simulink model "mp_rl_load_class"  (R2021b)
settings: Solver=ode23tb  StartTime=0.0  StopTime=0.1  RelTol=1e-3
values from neighbouring files (symbols this model uses):
  A = -R/L    (= -200)    [init_mp_rl_load.m]    (also in init_mp_rl_load_class.m = 0.99)
  Atilde = -R/L    (= -1000)    [init_mp_rl_load_class.m]
  B = 1/L    (= 200)    [init_mp_rl_load.m]    (also in init_mp_rl_load_class.m = 0.01)
  Btilde = 1/L    (= 1000)    [init_mp_rl_load_class.m]
  C = 1    [init_mp_rl_load.m]    (also in init_mp_rl_load_class.m)
  i_ref_amp = 50    [init_mp_rl_load_class.m]
  i_ref_omega = 2*pi*50    (= 314.159265359)    [init_mp_rl_load_class.m]
  rho = 0    [init_mp_rl_load.m]    (also in init_mp_rl_load_class.m = 0.0001)
  ts = 1e-5    (= 1e-05)    [init_mp_rl_load_class.m]
  udc = 250    [init_mp_rl_load.m]    (also in init_mp_rl_load_class.m)
settings Model: Creator=dbagn  LastModifiedBy=dbagn
settings SolverCC: AlgebraicLoopSolver=TrustRegion
settings DebuggingCC: SFMachineParentedDataDiag=warning
settings SFSimCC: CustomCodeUndefinedFunction=UseInterfaceOnly

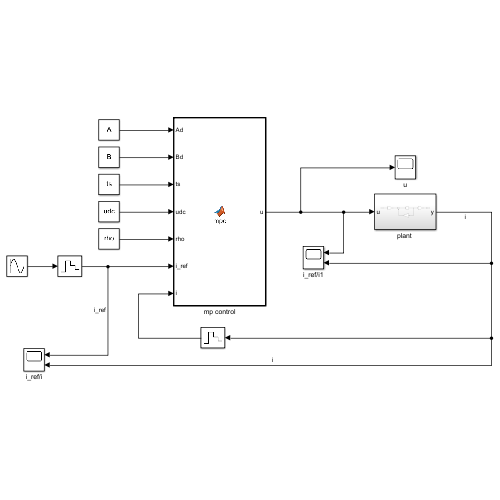
[thumbnail: Simulink's stored preview of the top-level diagram]
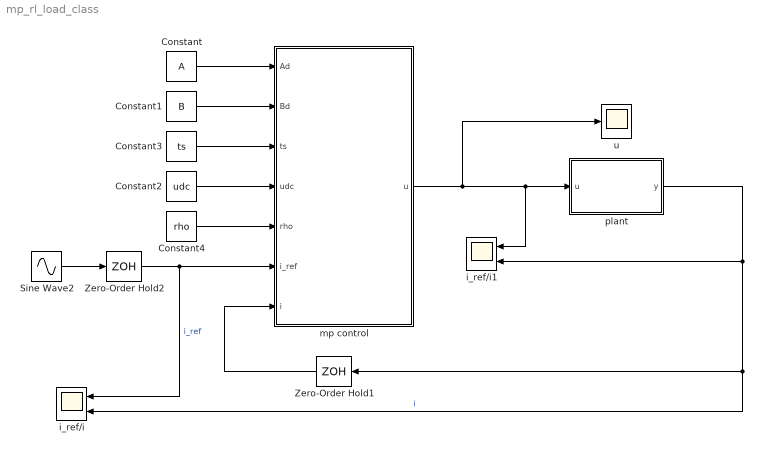
== system mp_rl_load_class ==
  Constant : Constant  Value=A
  Constant1 : Constant  Value=B
  Constant2 : Constant  Value=udc
  Constant3 : Constant  Value=ts
  Constant4 : Constant  Value=rho
  Sine Wave2 : Sin  Amplitude=i_ref_amp  Frequency=i_ref_omega  SampleTime=0
  Zero-Order Hold1 : ZeroOrderHold  SampleTime=ts
  Zero-Order Hold2 : ZeroOrderHold  SampleTime=ts
  i_ref/i : Scope  NumInputPorts=2
  i_ref/i1 : Scope  NumInputPorts=2
  mp control : MATLAB Function  TreatAsAtomicUnit=on  SystemSampleTime=ts
  "plant " : Subsystem
  u : Scope
  wires:
  mp control/1(u) -> u/1, "plant "/1(u), i_ref/i1/1
  Sine Wave2/1 -> Zero-Order Hold2/1
  Zero-Order Hold2/1 -> i_ref/i/1, mp control/6(i_ref)  "i_ref"
  "plant "/1(y) -> Zero-Order Hold1/1, i_ref/i/2, i_ref/i1/2  "i"
  Zero-Order Hold1/1 -> mp control/7(i)
  Constant/1 -> mp control/1(Ad)
  Constant1/1 -> mp control/2(Bd)
  Constant2/1 -> mp control/4(udc)
  Constant3/1 -> mp control/3(ts)
  Constant4/1 -> mp control/5(rho)

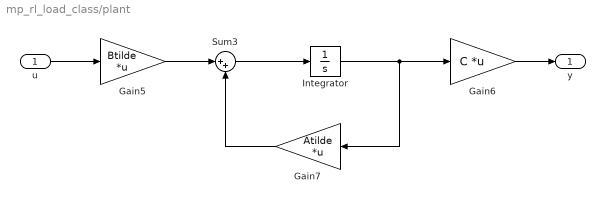
== system mp_rl_load_class/plant  ==
  u : Inport
  Gain5 : Gain  Gain=Btilde  Multiplication=Matrix(K*u)
  Gain6 : Gain  Gain=C  Multiplication=Matrix(K*u)
  Gain7 : Gain  Gain=Atilde  Multiplication=Matrix(K*u)
  Integrator : Integrator
  Sum3 : Sum  Inputs=|++
  y : Outport
  wires:
  Sum3/1 -> Integrator/1
  Gain7/1 -> Sum3/2
  u/1 -> Gain5/1
  Gain5/1 -> Sum3/1
  Gain6/1 -> y/1
  Integrator/1 -> Gain7/1, Gain6/1

== matlab function mp_rl_load_class/mp control ==
  data: Ad input; u output; Bd input; ts input; udc input; rho input; i_ref input; i input
function u = mpc(Ad, Bd, ts, udc, rho, i_ref, i)

persistent u_z

if isempty(u_z)
    u_z = 0;
end

    if (u_z == 0)
        i_hat_1 = Ad*i+Bd*udc; % u = udc
        i_hat_2 = Ad*i; % u = 0
        i_hat_3 = Ad*i-Bd*udc; % u = -udc
    
        J1 = (i_ref - i_hat_1)^2+rho*(udc-u_z)^2;
        J2 = (i_ref - i_hat_2)^2+rho*(0-u_z)^2;
        J3 = (i_ref - i_hat_3)^2+rho*(-udc-u_z)^2;
    
        if ((J1 <= J2) && (J1 <= J3))
            u = udc;
        elseif ((J2 <= J1) && (J2 <= J3))
            u = 0;
        else 
            u = -udc;
        end
    elseif (u_z == udc)
        i_hat_1 = Ad*i+Bd*udc; % u = udc
        i_hat_2 = Ad*i; % u = 0
    
        J1 = (i_ref - i_hat_1)^2+rho*(udc-u_z)^2; % 
        J2 = (i_ref - i_hat_2)^2+rho*(0-u_z)^2;
        
        if (J1 <= J2)
            u = udc;
        else
            u = 0;
        end
    else
        i_hat_2 = Ad*i; % u = 0
        i_hat_3 = Ad*i-Bd*udc; % u = -udc
    
        J2 = (i_ref - i_hat_2)^2+rho*(0-u_z)^2; % u(k) =0
        J3 = (i_ref - i_hat_3)^2+rho*(-udc-u_z)^2; % u(k) = -udc
    
        if (J2 <= J3)
            u = 0;
        else
            u = -udc;
        end
    end
u_z = u;
end
